simulink library "Chassis_Alpha"  (R2013b)
settings: Solver=ode45  StartTime=0.0  StopTime=10.0  RelTol=1e-3
undefined symbols (not defined in the file or in its folder): Chassis, lat0, lon0, open_system, Suspension, transMatrix, v_ds, X, xx_ds, Y, yy_ds, Z
libraries: Chassis_Alpha x8, sm_lib x8, simulink x4, nesl_utility x3, vrlib x1
Description:
  | Copyright 2013-2014 The MathWorks, Inc.
settings Model: Creator=mbrauer  LastModifiedBy=mbrauer

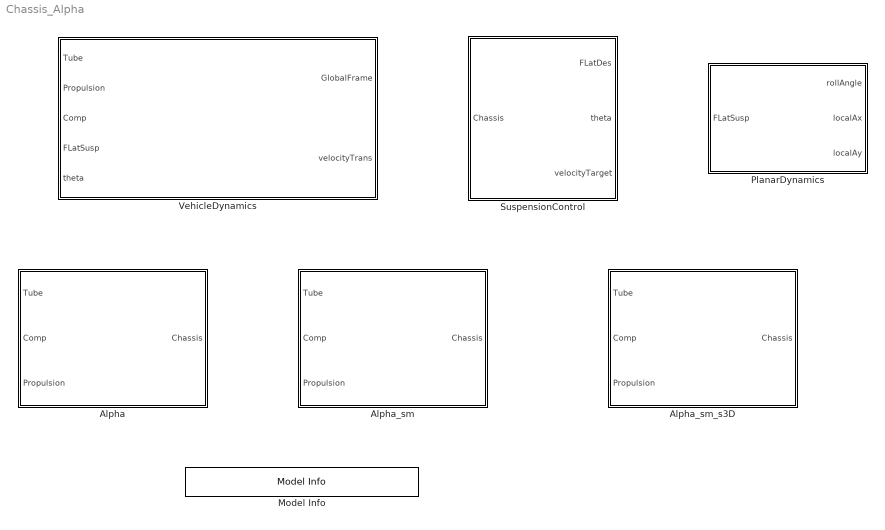
== system Chassis_Alpha ==
  Alpha : Subsystem
  Alpha_sm : Subsystem
  Alpha_sm_s3D : Subsystem  InitFcn=open_system([gcb,'/VR Sink'])
  Model Info : simulink/Model-Wide Utilities/Model Info  InitialBlockCM=None  BlockCM=none  Frame=on  DisplayStringWithTags=%<Description>  HorizontalTextAlignment=Center  LeftAlignmentValue=0.5  SourceBlockDiagram=Chassis_Alpha  TagMaxNumber=20
  PlanarDynamics : Subsystem
  SuspensionControl : Subsystem
  VehicleDynamics : Subsystem

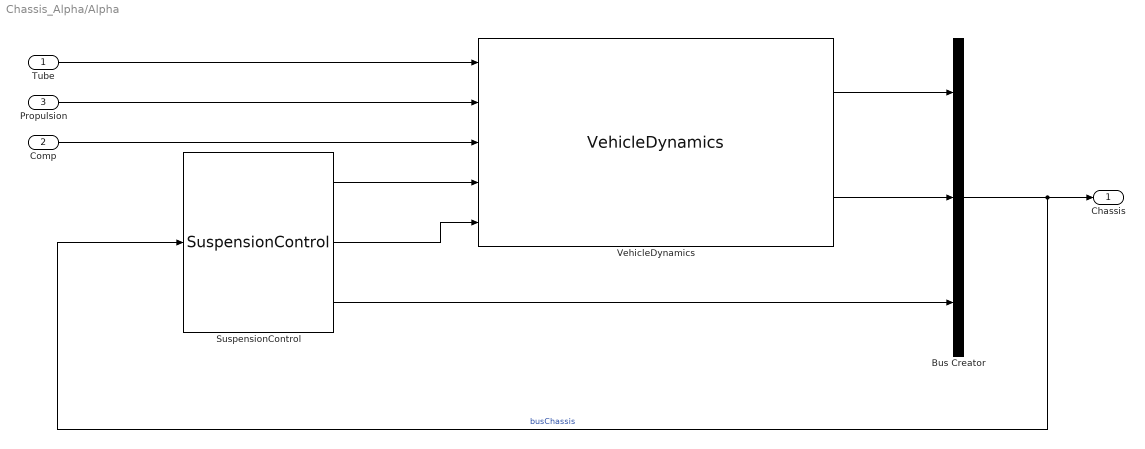
== system Chassis_Alpha/Alpha ==
  "Tube " : Inport
  Comp : Inport  Port=2
  Propulsion : Inport  Port=3
  Bus Creator : BusCreator  Inputs=3  NonVirtualBus=on
  SuspensionControl : Chassis_Alpha/SuspensionControl
  VehicleDynamics : Chassis_Alpha/VehicleDynamics
  Chassis : Outport
  wires:
  Bus Creator/1 -> SuspensionControl/1, Chassis/1  "busChassis"
  Comp/1 -> VehicleDynamics/3
  "Tube "/1 -> VehicleDynamics/1
  VehicleDynamics/1 -> Bus Creator/1
  VehicleDynamics/2 -> Bus Creator/2
  Propulsion/1 -> VehicleDynamics/2
  SuspensionControl/1 -> VehicleDynamics/4
  SuspensionControl/2 -> VehicleDynamics/5
  SuspensionControl/3 -> Bus Creator/3

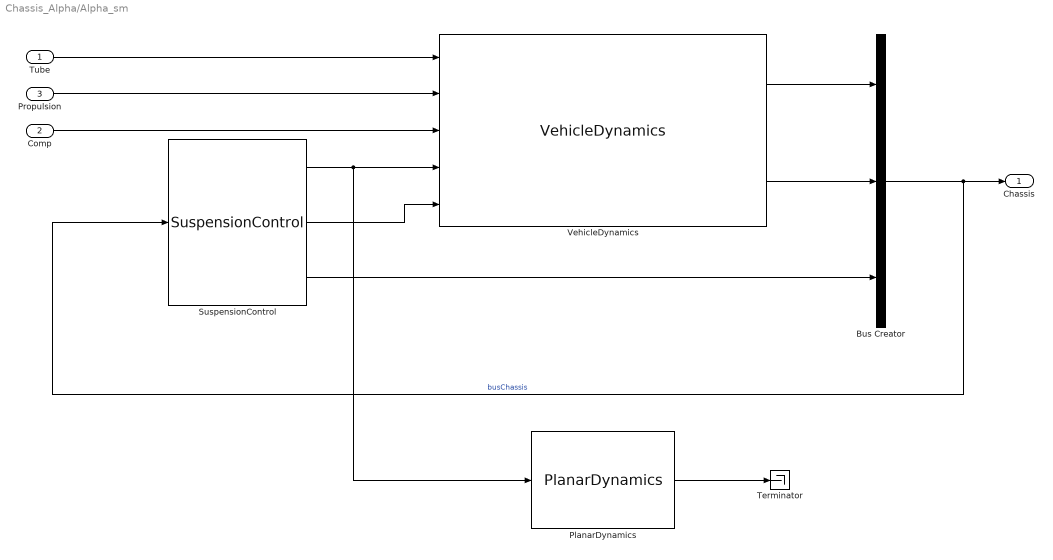
== system Chassis_Alpha/Alpha_sm ==
  "Tube " : Inport
  Comp : Inport  Port=2
  Propulsion : Inport  Port=3
  Bus Creator : BusCreator  Inputs=3  NonVirtualBus=on
  PlanarDynamics : Chassis_Alpha/PlanarDynamics
  SuspensionControl : Chassis_Alpha/SuspensionControl
  Terminator : Terminator
  VehicleDynamics : Chassis_Alpha/VehicleDynamics
  Chassis : Outport
  wires:
  SuspensionControl/3 -> Bus Creator/3
  SuspensionControl/2 -> VehicleDynamics/5
  SuspensionControl/1 -> PlanarDynamics/1, VehicleDynamics/4
  Propulsion/1 -> VehicleDynamics/2
  VehicleDynamics/2 -> Bus Creator/2
  VehicleDynamics/1 -> Bus Creator/1
  "Tube "/1 -> VehicleDynamics/1
  Comp/1 -> VehicleDynamics/3
  Bus Creator/1 -> Chassis/1, SuspensionControl/1  "busChassis"
  PlanarDynamics/1 -> Terminator/1

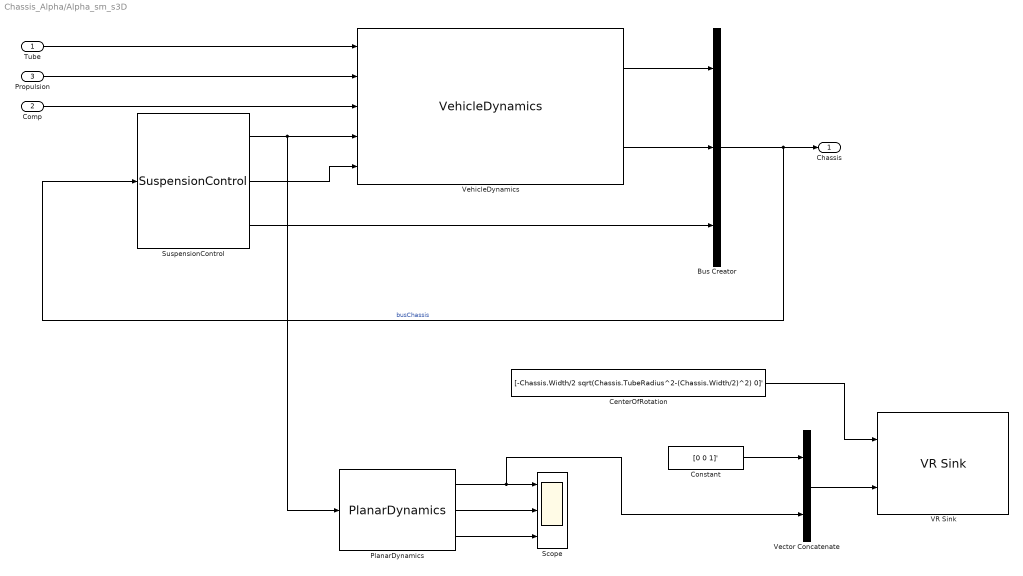
== system Chassis_Alpha/Alpha_sm_s3D ==
  "Tube " : Inport
  Comp : Inport  Port=2
  Propulsion : Inport  Port=3
  Bus Creator : BusCreator  Inputs=3  NonVirtualBus=on
  CenterOfRotation : Constant  Value=[-Chassis.Width/2 sqrt(Chassis.TubeRadius^2-(Chassis.Width/2)^2) 0]'
  Constant : Constant  Value=[0 0 1]'
  PlanarDynamics : Chassis_Alpha/PlanarDynamics
  Scope : Scope  NumInputPorts=3
      settings: YMin=-0.5~-0.1~-0.35  YMax=0.4~0.125~0.2  Decimation=10
  SuspensionControl : Chassis_Alpha/SuspensionControl
  VR Sink : vrlib/VR Sink  InstantiateOnLoad=on  SampleTime=0.1  ViewEnable=on  RemoteChange=off  RemoteView=off  FieldsWritten=HyperPod.center.3.1.1.double#HyperPod.rotation.4.1.1.double  WorldFileName=hyperLoopPod3D.wrl  AutoView=off  VideoDimensions=[]  AllowVariableSize=off
  Vector Concatenate : Concatenate
  VehicleDynamics : Chassis_Alpha/VehicleDynamics
  Chassis : Outport
  wires:
  PlanarDynamics/3 -> Scope/3
  PlanarDynamics/2 -> Scope/2
  Vector Concatenate/1 -> VR Sink/2
  CenterOfRotation/1 -> VR Sink/1
  Constant/1 -> Vector Concatenate/1
  PlanarDynamics/1 -> Scope/1, Vector Concatenate/2
  Bus Creator/1 -> SuspensionControl/1, Chassis/1  "busChassis"
  Comp/1 -> VehicleDynamics/3
  "Tube "/1 -> VehicleDynamics/1
  VehicleDynamics/1 -> Bus Creator/1
  VehicleDynamics/2 -> Bus Creator/2
  Propulsion/1 -> VehicleDynamics/2
  SuspensionControl/1 -> PlanarDynamics/1, VehicleDynamics/4
  SuspensionControl/2 -> VehicleDynamics/5
  SuspensionControl/3 -> Bus Creator/3

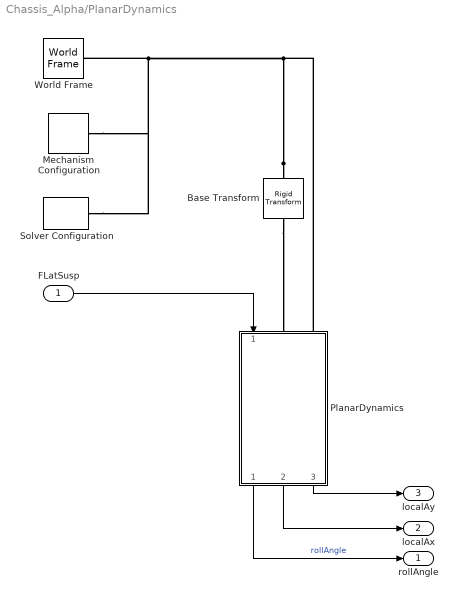
== system Chassis_Alpha/PlanarDynamics ==
  FLatSusp : Inport
  Base Transform : sm_lib/Frames and Transforms/Rigid Transform  TranslationMethod=None  TranslationLengthUnit=m  TranslationStandardAxis=+Z  TranslationStandardOffset=0  TranslationCartesianOffset=[0 0 0]  TranslationROffset=0  TranslationROffsetUnits=m  TranslationZOffset=0  TranslationZOffsetUnits=m  TranslationThetaOffset=0  TranslationThetaOffsetUnits=deg  RotationMethod=AlignedAxes  RotationAngleUnits=deg  RotationStandardAxis=+Z  RotationAngle=0  RotationArbitraryAxis=[0 0 1]  FollAlignAxisA=+Z  BaseAlignAxisA=-Y  FollAlignAxisB=+Y  BaseAlignAxisB=+X  BlockFunction=simmechanics.library.frames_transforms.rigid_transform
  Mechanism Configuration : sm_lib/Utilities/Mechanism Configuration  GravityVector=[0 0 -9.81]  GravityUnits=m/s^2  AllowGravitySignal=off  LinearizationDelta=0.001  BlockFunction=simmechanics.library.utilities.mechanism_configuration
  PlanarDynamics : Subsystem  mask(Upper Link){R=Chassis.TubeRadius, cH=Chassis.Height, cW=Chassis.Width, M=Chassis.Mass, D=5e3 % magic number}
      mask prompts: R "Tube Radius (m)"; cH "Chass height (m):"; cW "Chassis width (m):"; M "Chassis mass (kg)"; D "Damping (N/rad/s)"
      mask help: Upper link of the double pendulum mechanism
      mask init:
      | % Solve trigonmetry to determine chassis location.
      | % Assumes point contact at bottom edges with tube.
      | Alpha  = sqrt(R^2-(cW/2)^2);
      | AirGap = R-Alpha;
  Solver Configuration : nesl_utility/Solver Configuration  PhysicalDomain=network_engine_domain  SubClassName=solver  LeftPortType=input  RightPortType=generic  Accelerate=off  Tones=[]  Harmonics=[]  SimulateNoise=off  Profile=off  UseLocalSampling=off  EnableSwitchedLinearOptims=on  FrequencyDomain=off  UseCCode=off  RelTol=0.001  AbsTol=1e-06  MinStep=1e-09  ToWorkspace=off  DoDC=off  ResidualTolerance=1e-9  UseLocalSolver=off  LocalSolverChoice=NE_BACKWARD_EULER_ADVANCER  LocalSolverSampleTime=.001  DoFixedCost=off  MaxNonlinIter=3  MaxModeIter=2  LinearAlgebra=Sparse  DelaysMemoryBudget=1024
  World Frame : sm_lib/Frames and Transforms/World Frame  BlockFunction=simmechanics.library.frames_transforms.world_frame
  rollAngle : Outport
  localAx : Outport  Port=2
  localAy : Outport  Port=3
  wires:
  PlanarDynamics/3(localAy) -> localAy/1
  PlanarDynamics/2(localAx) -> localAx/1
  FLatSusp/1 -> PlanarDynamics/1(FLatSusp)
  PlanarDynamics/1(rollAngle) -> rollAngle/1  "rollAngle"
  connections:
  Base Transform/LConn1 -- World Frame/RConn1 -- Mechanism Configuration/RConn1 -- Solver Configuration/RConn1 -- PlanarDynamics/LConn2
  Base Transform/RConn1 -- PlanarDynamics/LConn1

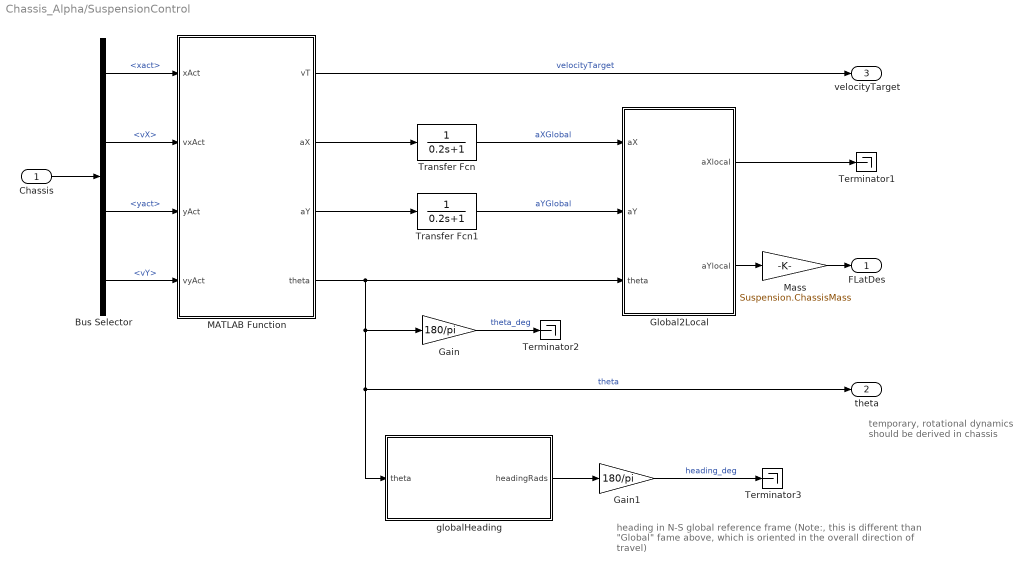
== system Chassis_Alpha/SuspensionControl ==
  note: temporary, rotational dynamics
      | should be derived in chassis
  note: heading in N-S global reference frame
      | (Note:, this is different than "Global" fame above, which is oriented
      | in the overall direction of travel)
  Chassis : Inport
  Bus Selector : BusSelector  OutputSignals=GlobalFrame.xact,GlobalFrame.vX,GlobalFrame.yact,GlobalFrame.vY
  Gain : Gain  Gain=180/pi
  Gain1 : Gain  Gain=180/pi
  Global2Local : MATLAB Function  TreatAsAtomicUnit=on
  MATLAB Function : MATLAB Function  TreatAsAtomicUnit=on
  Mass : Gain  Gain=Suspension.ChassisMass
  Terminator1 : Terminator
  Terminator2 : Terminator
  Terminator3 : Terminator
  Transfer Fcn : TransferFcn  Denominator=[0.2 1]
  Transfer Fcn1 : TransferFcn  Denominator=[0.2 1]
  globalHeading : MATLAB Function  TreatAsAtomicUnit=on
  FLatDes : Outport
  theta : Outport  Port=2
  velocityTarget : Outport  Port=3
  wires:
  Gain1/1 -> Terminator3/1  "heading_deg"
  globalHeading/1(headingRads) -> Gain1/1
  MATLAB Function/2(aX) -> Transfer Fcn/1
  MATLAB Function/3(aY) -> Transfer Fcn1/1
  Transfer Fcn/1 -> Global2Local/1(aX)  "aXGlobal"
  Transfer Fcn1/1 -> Global2Local/2(aY)  "aYGlobal"
  Gain/1 -> Terminator2/1  "theta_deg"
  MATLAB Function/4(theta) -> Gain/1, theta/1, globalHeading/1(theta), Global2Local/3(theta)  "theta"
  Chassis/1 -> Bus Selector/1
  Bus Selector/2 -> MATLAB Function/2(vxAct)  "<vX>"
  Bus Selector/1 -> MATLAB Function/1(xAct)  "<xact>"
  Bus Selector/3 -> MATLAB Function/3(yAct)  "<yact>"
  Bus Selector/4 -> MATLAB Function/4(vyAct)  "<vY>"
  Global2Local/1(aXlocal) -> Terminator1/1
  Global2Local/2(aYlocal) -> Mass/1
  Mass/1 -> FLatDes/1
  MATLAB Function/1(vT) -> velocityTarget/1  "velocityTarget"

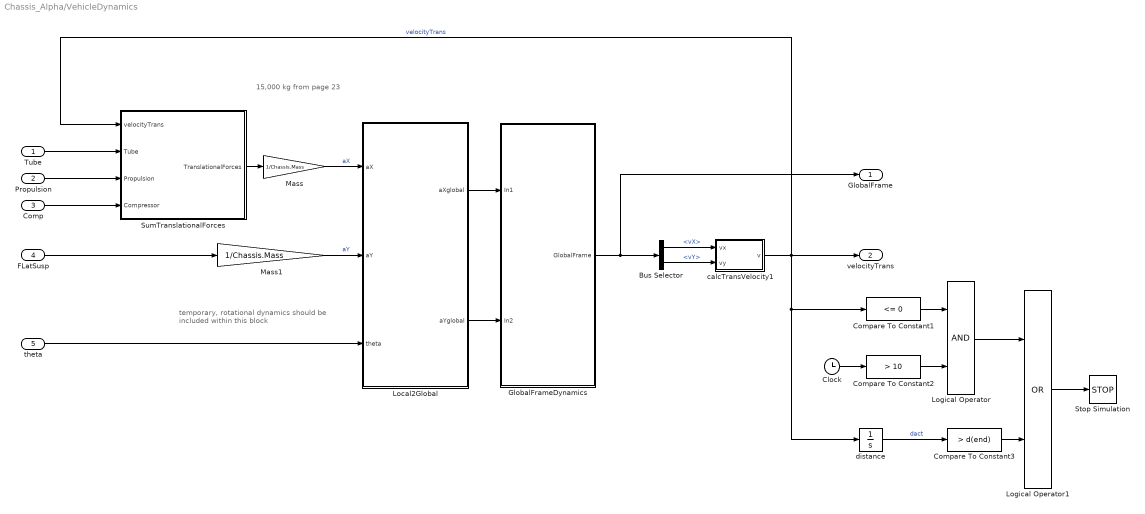
== system Chassis_Alpha/VehicleDynamics ==
  note: 15,000 kg from page 23
  note: temporary, rotational dynamics should
      | be included within this block
  "Tube " : Inport
  Propulsion : Inport  Port=2
  Comp : Inport  Port=3
  FLatSusp : Inport  Port=4
  theta : Inport  Port=5
  Bus Selector : BusSelector  OutputSignals=vX,vY
  Clock : Clock
  Compare To Constant1 : simulink/Logic and Bit Operations/Compare To Constant  relop=<=  const=0  OutDataTypeStr=boolean
  Compare To Constant2 : simulink/Logic and Bit Operations/Compare To Constant  relop=>  const=10  OutDataTypeStr=boolean  ZeroCross=off
  Compare To Constant3 : simulink/Logic and Bit Operations/Compare To Constant  relop=>  const=d(end)  OutDataTypeStr=boolean  ZeroCross=off
  GlobalFrameDynamics : Subsystem
  Local2Global : MATLAB Function  TreatAsAtomicUnit=on
  Logical Operator : Logic  AllPortsSameDT=off  OutDataTypeStr=boolean
  Logical Operator1 : Logic  Operator=OR  AllPortsSameDT=off  OutDataTypeStr=boolean
  Mass : Gain  Gain=1/Chassis.Mass
  Mass1 : Gain  Gain=1/Chassis.Mass
  Stop Simulation : Stop
  SumTranslationalForces : Subsystem
  calcTransVelocity1 : MATLAB Function  TreatAsAtomicUnit=on
  distance : Integrator
  GlobalFrame : Outport
  velocityTrans : Outport  Port=2
  wires:
  Bus Selector/2 -> calcTransVelocity1/2(vy)  "<vY>"
  Bus Selector/1 -> calcTransVelocity1/1(vx)  "<vX>"
  GlobalFrameDynamics/1(GlobalFrame) -> Bus Selector/1, GlobalFrame/1
  Local2Global/2(aYglobal) -> GlobalFrameDynamics/2(In2)
  Local2Global/1(aXglobal) -> GlobalFrameDynamics/1(In1)
  Compare To Constant3/1 -> Logical Operator1/2
  Logical Operator/1 -> Logical Operator1/1
  Logical Operator1/1 -> Stop Simulation/1
  Compare To Constant2/1 -> Logical Operator/2
  Clock/1 -> Compare To Constant2/1
  Compare To Constant1/1 -> Logical Operator/1
  distance/1 -> Compare To Constant3/1  "dact"
  "Tube "/1 -> SumTranslationalForces/2("Tube ")
  Propulsion/1 -> SumTranslationalForces/3(Propulsion)
  Comp/1 -> SumTranslationalForces/4(Compressor)
  Mass1/1 -> Local2Global/2(aY)  "aY"
  Mass/1 -> Local2Global/1(aX)  "aX"
  FLatSusp/1 -> Mass1/1
  SumTranslationalForces/1(TranslationalForces) -> Mass/1
  calcTransVelocity1/1(v) -> distance/1, Compare To Constant1/1, velocityTrans/1, SumTranslationalForces/1(velocityTrans)  "velocityTrans"
  theta/1 -> Local2Global/3(theta)

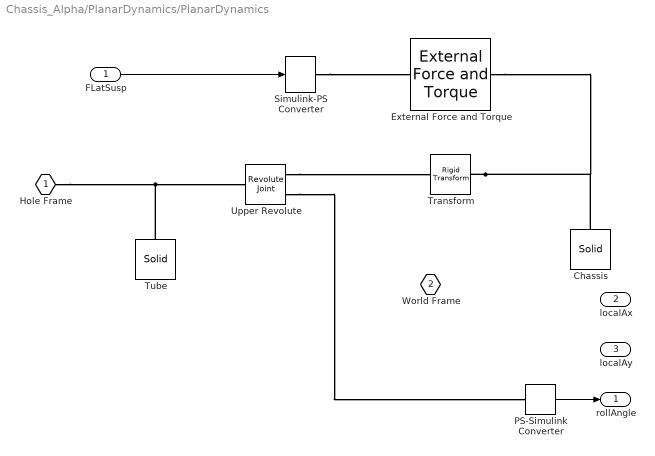
== system Chassis_Alpha/PlanarDynamics/PlanarDynamics ==
  FLatSusp : Inport
  Chassis : sm_lib/Body Elements/Solid  InertiaType=PointMass  Mass=M  MassUnits=kg  CenterOfMass=[0 0 0]  CenterOfMassUnits=m  MomentsOfInertia=[1 1 1]  MomentsOfInertiaUnits=kg*m^2  ProductsOfInertia=[0 0 0]  ProductsOfInertiaUnits=kg*m^2  DensityBased=on  Density=1  DensityUnits=kg/m^3  GraphicType=FromGeometry  MarkerShape=Sphere  MarkerSize=1  MarkerSizeUnits=m  GraphicVisPropType=SimpleVisualProperties  GraphicDiffuseColor=[0.2 0.4 1.0]  GraphicSpecularColor=[0.2 0.2 0.2]  GraphicAmbientColor=[0.5 0.5 0.5]  GraphicEmissiveColor=[0.1 0.1 0.1]  GraphicShininess=24.0  GraphicOpacity=1  GeometryShape=Brick  RectangleSize=[1 1]  RectangleSizeUnits=m  BrickDimensions=[cH cW 1]  BrickDimensionUnits=m  CylinderRadius=1  CylinderRadiusUnits=cm  CylinderLength=1  CylinderLengthUnits=cm  SphereRadius=1  SphereRadiusUnits=m  EllipsoidRadii=[1 1 1]  EllipsoidRadiiUnits=m  ExtrusionCrossSection=[1 1; -1 1; -1 -1; 1 -1]  ExtrusionCrossSectionUnits=m  ExtrusionLength=1  ExtrusionLengthUnits=m  PolygonNumSides=1  PolygonOuterRadius=1  PolygonOuterRadiusUnits=m  ExtGeomFileUnits=m  RevolutionCrossSection=[1 1; 1 -1; 2 -1; 2 1]  RevolutionCrossSectionUnits=m  RevolutionExtent=Full  RevolutionAngle=180  RevolutionAngleUnits=deg  BlockFunction=simmechanics.library.body_elements.solid
  External Force and Torque : sm_lib/Forces and Torques/External Force and Torque  ForceResolutionFrame=World  EnableForceX=on  EnableForceY=off  EnableForceZ=off  EnableForce=off  TorqueResolutionFrame=AttachedFrame  EnableTorqueX=off  EnableTorqueY=off  EnableTorqueZ=off  EnableTorque=off  BlockFunction=simmechanics.library.forces_torques.external_force_torque
  PS-Simulink Converter : nesl_utility/PS-Simulink Converter  PhysicalDomain=network_engine_domain  SubClassName=ps_output  LeftPortType=input  RightPortType=output  PseudoPeriodic=off  Frequencies=[]  Unit=1  AffineConversion=off
  Simulink-PS Converter : nesl_utility/Simulink-PS Converter  PhysicalDomain=network_engine_domain  SubClassName=ps_input  LeftPortType=input  RightPortType=output  PseudoPeriodic=off  Frequencies=[]  NoiseDistribution=none  NoiseParameters=[]  Unit=N  AffineConversion=off  InputFiltering=off  SimscapeFilterOrder=1  InputFilterTimeConstant=0.001  UdotUserProvided=1
  Transform : sm_lib/Frames and Transforms/Rigid Transform  TranslationMethod=Cartesian  TranslationLengthUnit=m  TranslationStandardAxis=+Z  TranslationStandardOffset=0  TranslationCartesianOffset=[R-AirGap-cH/2 0 0]  TranslationROffset=0  TranslationROffsetUnits=m  TranslationZOffset=0  TranslationZOffsetUnits=m  TranslationThetaOffset=0  TranslationThetaOffsetUnits=deg  RotationMethod=None  RotationAngleUnits=deg  RotationStandardAxis=+Z  RotationAngle=0  RotationArbitraryAxis=[0 0 1]  FollAlignAxisA=+X  BaseAlignAxisA=+Y  FollAlignAxisB=+Y  BaseAlignAxisB=+Z  BlockFunction=simmechanics.library.frames_transforms.rigid_transform
  Tube : sm_lib/Body Elements/Solid  InertiaType=PointMass  Mass=1  MassUnits=kg  CenterOfMass=[0 0 0]  CenterOfMassUnits=m  MomentsOfInertia=[1 1 1]  MomentsOfInertiaUnits=kg*m^2  ProductsOfInertia=[0 0 0]  ProductsOfInertiaUnits=kg*m^2  DensityBased=on  Density=1  DensityUnits=kg/m^3  GraphicType=FromGeometry  MarkerShape=Sphere  MarkerSize=1  MarkerSizeUnits=m  GraphicVisPropType=SimpleVisualProperties  GraphicDiffuseColor=[0.6 0.6 0.6]  GraphicSpecularColor=[0.2 0.2 0.2]  GraphicAmbientColor=[0.5 0.5 0.5]  GraphicEmissiveColor=[0.1 0.1 0.1]  GraphicShininess=24.0  GraphicOpacity=1  GeometryShape=Cylinder  RectangleSize=[1 1]  RectangleSizeUnits=m  BrickDimensions=[cW cH 1]  BrickDimensionUnits=m  CylinderRadius=R  CylinderRadiusUnits=m  CylinderLength=1  CylinderLengthUnits=cm  SphereRadius=1  SphereRadiusUnits=m  EllipsoidRadii=[1 1 1]  EllipsoidRadiiUnits=m  ExtrusionCrossSection=[1 1; -1 1; -1 -1; 1 -1]  ExtrusionCrossSectionUnits=m  ExtrusionLength=1  ExtrusionLengthUnits=m  PolygonNumSides=1  PolygonOuterRadius=1  PolygonOuterRadiusUnits=m  ExtGeomFileUnits=m  RevolutionCrossSection=[1 1; 1 -1; 2 -1; 2 1]  RevolutionCrossSectionUnits=m  RevolutionExtent=Full  RevolutionAngle=180  RevolutionAngleUnits=deg  BlockFunction=simmechanics.library.body_elements.solid
  Upper Revolute : sm_lib/Joints/Revolute Joint  SenseConstraintForceX=off  SenseConstraintForceY=off  SenseConstraintForceZ=off  SenseConstraintTorqueX=off  SenseConstraintTorqueY=off  SenseConstraintTorqueZ=off  ConstraintWrenchDir=FollowerOnBase  ConstraintWrenchFrame=BaseFrame  EquilibriumPosition=0  EquilibriumPositionUnits=rad  SpringStiffness=0  SpringStiffnessUnits=N*m/rad  DampingCoefficient=D  DampingCoefficientUnits=N*m/(rad/s)  TorqueActuationMode=NoTorque  MotionActuationMode=ComputedMotion  SensePosition=on  SenseVelocity=off  SenseAcceleration=off  SenseTorqueForce=off  PositionTargetValue=0  PositionTargetValueUnits=deg  PositionTargetSpecify=on  PositionTargetPriority=High  VelocityTargetValue=0  VelocityTargetValueUnits=rad/s  VelocityTargetSpecify=off  VelocityTargetPriority=Low  BlockFunction=simmechanics.library.joints.revolute_joint
  Hole Frame : PMIOPort  Port=1  Side=Left
  World Frame : PMIOPort  Port=2  Side=Left
  rollAngle : Outport
  localAx : Outport  Port=2
  localAy : Outport  Port=3
  wires:
  ? -> localAy/1
  ? -> localAx/1
  FLatSusp/1 -> Simulink-PS Converter/1
  PS-Simulink Converter/1 -> rollAngle/1
  connections:
  Hole Frame/RConn1 -- Tube/RConn1 -- Upper Revolute/LConn1
  Upper Revolute/RConn1 -- Transform/LConn1
  Transform/RConn1 -- Chassis/RConn1 -- External Force and Torque/RConn1
  Simulink-PS Converter/RConn1 -- External Force and Torque/LConn1
  Upper Revolute/RConn2 -- PS-Simulink Converter/LConn1

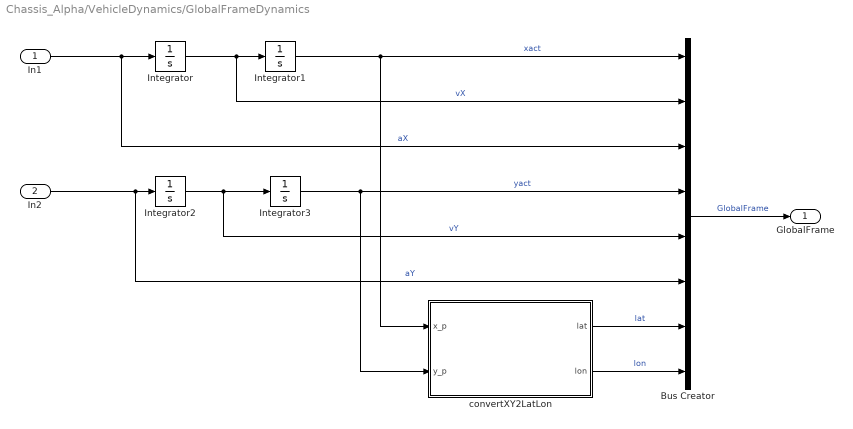
== system Chassis_Alpha/VehicleDynamics/GlobalFrameDynamics ==
  In1 : Inport
  In2 : Inport  Port=2
  Bus Creator : BusCreator  Inputs=8
  Integrator{,1..3} (4 alike) : Integrator
  convertXY2LatLon : MATLAB Function  TreatAsAtomicUnit=on
  GlobalFrame : Outport
  wires:
  convertXY2LatLon/2(lon) -> Bus Creator/8  "lon"
  convertXY2LatLon/1(lat) -> Bus Creator/7  "lat"
  Bus Creator/1 -> GlobalFrame/1  "GlobalFrame"
  Integrator2/1 -> Integrator3/1, Bus Creator/5  "vY"
  In1/1 -> Integrator/1, Bus Creator/3  "aX"
  Integrator3/1 -> Bus Creator/4, convertXY2LatLon/2(y_p)  "yact"
  Integrator1/1 -> Bus Creator/1, convertXY2LatLon/1(x_p)  "xact"
  In2/1 -> Integrator2/1, Bus Creator/6  "aY"
  Integrator/1 -> Integrator1/1, Bus Creator/2  "vX"

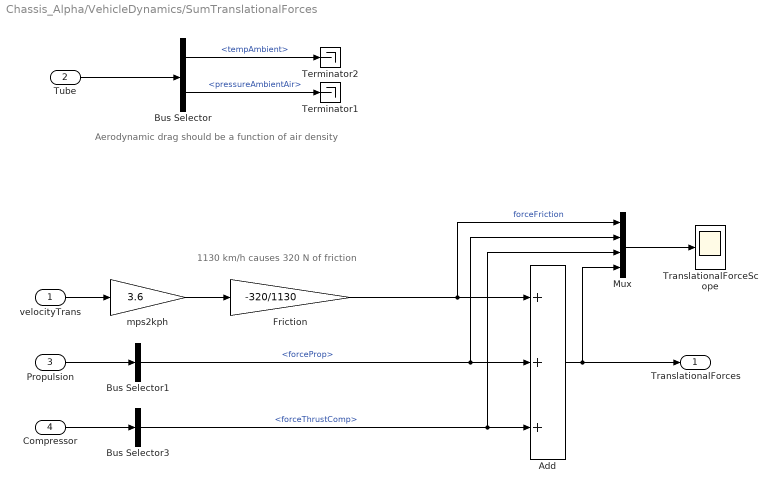
== system Chassis_Alpha/VehicleDynamics/SumTranslationalForces ==
  note: 1130 km/h causes 320 N of friction
  note: Aerodynamic drag should be a function of air density
  velocityTrans : Inport
  "Tube " : Inport  Port=2
  Propulsion : Inport  Port=3
  Compressor : Inport  Port=4
  Add : Sum  Inputs=+++
  Bus Selector : BusSelector  OutputSignals=tempAmbient,pressureAmbientAir
  Bus Selector1 : BusSelector  OutputSignals=forceProp
  Bus Selector3 : BusSelector  OutputSignals=forceThrustComp
  Friction : Gain  Gain=-320/1130
  Mux : Mux
  Terminator1 : Terminator
  Terminator2 : Terminator
  TranslationalForceScope : Scope
  mps2kph : Gain  Gain=3.6
  TranslationalForces : Outport
  wires:
  Friction/1 -> Add/1, Mux/1  "forceFriction"
  Add/1 -> Mux/4, TranslationalForces/1
  Mux/1 -> TranslationalForceScope/1
  Bus Selector3/1 -> Add/3, Mux/3  "<forceThrustComp>"
  Bus Selector1/1 -> Add/2, Mux/2  "<forceProp>"
  Compressor/1 -> Bus Selector3/1
  Propulsion/1 -> Bus Selector1/1
  mps2kph/1 -> Friction/1
  Bus Selector/2 -> Terminator1/1  "<pressureAmbientAir>"
  Bus Selector/1 -> Terminator2/1  "<tempAmbient>"
  "Tube "/1 -> Bus Selector/1
  velocityTrans/1 -> mps2kph/1

== matlab function Chassis_Alpha/VehicleDynamics/GlobalFrameDynamics/convertXY2LatLon ==
  data: x_p input; lat output; y_p input; transMatrix parameter; lat0 parameter; lon0 parameter; lon output
function [lat, lon ] = convertXY2LatLon(x_p,y_p,transMatrix,lat0,lon0)
%reorientXY2LatLon  re-orient a single cartesian data point to latitude 
% and longitude in degrees. The translation matrix, which was used 
% to do the opposite conversion, is required.
%
%   Copyright 2013 - 2014 The MathWorks, Inc

%% Re-orient based on original transMatrix
x_y_p   = [x_p';y_p'];
x_y     = transMatrix\x_y_p;
x_p     = x_y(1,:)';
y_p     = x_y(2,:)';

%% Convert cartesian coordinates to latitude and longitude 
lat2met = 110958.98;    % one degree of latitude is 110958.98 m at 36 deg
lon2met = 90163.66;     % one degree of longitude is 90163.66 m at 36 deg

lon     = x_p/lon2met+lon0;
lat     = y_p/lat2met+lat0;

== matlab function Chassis_Alpha/SuspensionControl/Global2Local ==
  data: aX input; aY input; theta input; aXlocal output; aYlocal output
function [aXlocal, aYlocal]  = global2Local(aX,aY, theta)

transMatrix = [cos(theta) sin(theta);-sin(theta) cos(theta)];
aLocal      = transMatrix*[aX;aY];
aXlocal     = aLocal(1);
aYlocal     = aLocal(2);

== matlab function Chassis_Alpha/VehicleDynamics/Local2Global ==
  data: aX input; aY input; theta input; aXglobal output; aYglobal output
function [aXglobal, aYglobal]  = Local2Global(aX,aY, theta)

transMatrix     = [cos(theta) sin(theta);-sin(theta) cos(theta)];
transMatrixInv  = inv(transMatrix);
aGlobal         = transMatrixInv*[aX;aY];
aXglobal        = aGlobal(1);
aYglobal        = aGlobal(2);

== matlab function Chassis_Alpha/SuspensionControl/MATLAB Function ==
  data: vT output; xAct input; vxAct input; aX output; yAct input; vyAct input; xx_ds parameter; yy_ds parameter; v_ds parameter; aY output; theta output
function [vT, aX, aY, theta] = findIdealTraj(xAct, vxAct, yAct, vyAct, xx_ds, yy_ds, v_ds)
% determines the desired acceleration in x and y direction given an actual
% position (xAct, yAct) and velocity (vxAct, vyAct) with parameters of 
% ideal trajectory (xx_ds, yy_ds) and velocity (v_ds) profiles

%% Find index of next closest point in trajectory (not necessarily the closest)
% Find closest point
distToRouteX        = xx_ds - ones(size(xx_ds))*xAct;
distToRouteY        = yy_ds - ones(size(xx_ds))*yAct;
distToRoute         = sqrt(distToRouteX.^2+distToRouteY.^2);
[distToPoint, idxA] = min(distToRoute);   % idxA corresponds to closest point

% find next nearest point that isn't too close       
if idxA == 1
    idx = 2;                    % just getting started
elseif idxA == length(xx_ds)
    idx = idxA;        % last point
elseif distToPoint < 60; % if very close to the point, use the next point
    idx = idxA + 1;
else                % either the closest point or the point after it is next
    distToRoute_nearest = [distToRoute(idxA-1) distToRoute(idxA+1)]; 
    [~, idx_rel] = min(distToRoute_nearest);
    idx = idxA +idx_rel - 1; % idx_rel = 1, idx is idxA (next point is nearest)
                         % idx_rel = 2, idx is idxA + 1 (next point is after nearest)
end                   

if idx>length(xx_ds)
    error('index exceeds length of xx_ds')
end

%% Determine desired acceleration
% give default values for output values to make MATLAB happy
aX      = 0;
aY      = 0;
tau1    = [1;0];        
vT      = 0;

% Move target point out until necessary acelaration is below a limit
flagExtendView = true;

while flagExtendView

% Distance vector to next point
deltaX1 = xx_ds(idx) - xAct;
deltaY1 = yy_ds(idx) - yAct;
dist    = sqrt(deltaX1^2+deltaY1^2);
tau1    = [deltaX1;deltaY1];
tauNorm1= tau1/norm(tau1);

% Distance vector to point after next (to determine tanjential velocity at
% next point)
if idx == length(xx_ds)    % last point so just extend direction
    tauNorm2 = tauNorm1;    
else
    deltaX2 = xx_ds(idx+1) - xx_ds(idx);
    deltaY2 = yy_ds(idx+1) - yy_ds(idx);
    tau2    = [deltaX2;deltaY2];
    tauNorm2= tau2/norm(tau2);
end

% Velocity vector at next point
if and(any(isnan(tauNorm1)),any(isnan(tauNorm2)))
    vTemp = [1 1];  % this shouldn't happen
%     warning('duplicate route points found at index = %d',idx)
elseif any(isnan(tauNorm1))
    vTemp = tauNorm2;
elseif any(isnan(tauNorm2))
    vTemp = tauNorm1;
else
    vTemp   = mean([tauNorm1,tauNorm2],2); % take mean of direction vectors
end
vTemp   = vTemp/norm(vTemp);           % re-normalize (magnitude of 1)
vVec    = v_ds(idx)*vTemp;             % mutiply by velocity magnitude
vT      = sqrt(vVec(1)^2+vVec(2)^2);
      
% Acceleration      
vAct    = sqrt(vxAct^2+vyAct^2);       % current velocity magnitude
time    = 2*dist/(vAct+v_ds(idx));     % time to reach next point
aX      = (vVec(1) - vxAct)/time;   
aY      = (vVec(2) - vyAct)/time; 

if idx == length(xx_ds)  % last point, need to accept acceleration target
    flagExtendView = false;
elseif sqrt(aX^2+aY^2)>10
    idx = idx + 1; 
else
    flagExtendView = false;
end

end

%% Determine local orientation of vehicle
theta = atan2(tau1(2),tau1(1));

== matlab function Chassis_Alpha/VehicleDynamics/calcTransVelocity1 ==
  data: vx input; v output; vy input
function v = fcn(vx,vy)
v = (vx^2+vy^2)^0.5;

== matlab function Chassis_Alpha/SuspensionControl/globalHeading ==
  data: theta input; transMatrix parameter; headingRads output
function headingRads   = globalHeading(theta, transMatrix)

forwardLocal        = [1;0];
transMatrixLocal    = [cos(theta) sin(theta);-sin(theta) cos(theta)];
headingVector       = inv(transMatrix)*inv(transMatrixLocal)*forwardLocal;
headingRads         = atan2(headingVector(2),headingVector(1));
            % 0 deg is facing E. 
            % 90 is N
            % -90 is S
            % 180 or -180 is W
